simulink model "frft_qpsk_transceiver"  (R2025a)
settings: Solver=FixedStepDiscrete  StartTime=0.0  StopTime=1  RelTol=1e-3
PreLoadFcn:
  | % Add paths
  | addpath("dvb-s2/")
  | addpath("frft_filtering/")
  | addpath("gse")
  | 
  | 
  | 
  | 
  | setTxBurstLength = 10000;
  | txtmsg = ['Zynq radio HW/SW Co-design ÞÞÞÞ']; % Use only printable characters
  | 
  | %------------------------------------------------------------------------------------------------------
  | if ~isequal(size(txtmsg),[1 31])
  |     error('txtmsg must contain 31 characters');
  | end
  | 
  | [dataBits,msg] = zynqRadioHWSWQPSKgenHelloworldMsg(20); % generate 20 msgs for LUT
  | msgLUT = uint8(msg);
  | dataBitsLUT = dataBits(:);
  | Rsym                = 25e3;%1.92e6;
  | Config = zynqRadioHWSWQPSKTxRxParameters;
  | fs = Rsym*Config.SamplesPerSymbol;
  | word = [txtmsg newline];  % append a new line character to txtmsg
  | 
  | % The highest clock rate is 16 times the message character rate.
  | % As the message characters are fed at highest clock to FPGA
  | % repeat each character 16 times to maintain the message rate.
  | word = repelem(word.',16,1);
  | repeatTimes = ceil(setTxBurstLength/length(word));
  | inpData = complex(repmat(uint8(word),repeatTimes,1));
  | inUseTxBurstLength = length(inpData);
PostLoadFcn:
  | hScopeConfig = get_param([gcs '/HDL_QPSK/QPSK Tx Channel QPSK Rx/QPSK Rx/Frequency and Time Synchronizer/Symbol Synchronizer/No HDL/QPSK Receiver Eye Diagram'],'ScopeConfiguration');
  | hScopeConfig.OpenAtSimulationStart = false;
  | hScopeConfig.Visible = false;
  | clear hScopeConfig
InitFcn:
  | setTxBurstLength = 10000;
  | txtmsg = ['Zynq radio HW/SW Co-design ÞÞÞÞ']; % Use only printable characters
  | 
  | %------------------------------------------------------------------------------------------------------
  | if ~isequal(size(txtmsg),[1 31])
  |     error('txtmsg must contain 31 characters');
  | end
  | 
  | [dataBits,msg] = zynqRadioHWSWQPSKgenHelloworldMsg(20); % generate 20 msgs for LUT
  | msgLUT = uint8(msg);
  | dataBitsLUT = dataBits(:);
  | Rsym                = 25e3;%1.92e6;
  | Config = zynqRadioHWSWQPSKTxRxParameters;
  | fs = Rsym*Config.SamplesPerSymbol;
  | word = [txtmsg newline];  % append a new line character to txtmsg
  | 
  | % The highest clock rate is 16 times the message character rate.
  | % As the message characters are fed at highest clock to FPGA
  | % repeat each character 16 times to maintain the message rate.
  | word = repelem(word.',16,1);
  | repeatTimes = ceil(setTxBurstLength/length(word));
  | inpData = complex(repmat(uint8(word),repeatTimes,1));
  | inUseTxBurstLength = length(inpData);
undefined symbols (not defined in the file or in its folder): Add, dspblkCoreblockFVToolHelper, gcbh, Shift, unicode2native
libraries: hdlsllib x120, simulink x39, commseqgen3 x8, dsphdlsigops2 x4, whdledac x4, dsphdlfiltering2 x3, whdlutilities x3, dsphdlxfrm2 x2, dsphdlmathfun2 x2, commdigbbndpm3 x2, commchan3 x1, whdlmod x1
(part 2 of 5)

== system frft_qpsk_transceiver/Model Parameters/HDL_QPSK/QPSK Tx Channel QPSK Rx/QPSK Rx ==
  dataIn : Inport  OutDataTypeStr=fixdt(1,16,14)  PortDimensions=1  SampleTime=1/(Rsym*SamplesPerSymbol)
      settings: SignalType=complex
  validIn : Inport  Port=2  OutDataTypeStr=boolean  PortDimensions=1  SampleTime=1/(Rsym*SamplesPerSymbol)
  rstCS : Inport  Port=3  OutDataTypeStr=boolean  PortDimensions=1
      settings: SignalType=complex
  Automatic Gain Control : Subsystem  mask{Ref=AGCReference, LFG=AGCLoopGain}
      mask prompts: Ref "Error Detector Reference:"; LFG "Loop Filter Gain"
  Bus Creator : BusCreator  Inputs=4
  Bus Creator1 : BusCreator  Inputs=3
  Delay : Delay  DelayLength=1
  FRFT Interference Cancellation : Subsystem  Commented=on
      settings: PortSchema="{\"entries\":[{\"content\":{\"sides\":[{\"content\":{\"connectorIds\":[\"In1\",\"In2\"]},\"type\":\"ConnectorPlacement.EquallySpacedRectSide\",\"uuid\":\"50491e4b-448d-4897-93d5-82658af40e6a\"},{\"content\":{\"connectorIds\":[\"Out1\",\"Out2\"],\"side\":\"RIGHT\"},\"type\":\"ConnectorPlacement.EquallySpacedRectSide\",\"uuid\":\"92b7170a-fe32-477b-a0aa-07b62d03a88a\"},{\"content\":{\"connectorIds\":[\"In3\"],\"side\":\"TOP\"},\"type\":\"ConnectorPlacement.EquallySpacedRectSide\",\"uuid\":\"ae8eeabd-9a0c-434e-a24f-48ab553d0b87\"}]},\"type\":\"ConnectorPlacement.EquallySpacedConnector\",\"uuid\":\"9bc37ce9-ba4c-4d42-a736-75d3eb39cc46\"}],\"packageUris\":[\"http://schema.mathworks.com/mf0/Connector/R2020b\"],\"version\":\"1.0\"}"
  Frequency and Time Synchronizer : Subsystem
      settings: PortSchema="{\"entries\":[{\"content\":{\"sides\":[{\"content\":{\"connectorIds\":[\"In1\",\"In2\"]},\"type\":\"ConnectorPlacement.EquallySpacedRectSide\",\"uuid\":\"8bc6a452-5111-4806-8ca9-335cb622aea6\"},{\"content\":{\"connectorIds\":[\"Out1\",\"Out2\",\"Out3\",\"Out4\"],\"side\":\"RIGHT\"},\"type\":\"ConnectorPlacement.EquallySpacedRectSide\",\"uuid\":\"b0f43c98-f5c0-4f62-94ae-d69789942eef\"},{\"content\":{\"connectorIds\":[\"In3\",\"Out5\",\"Out6\"],\"side\":\"TOP\"},\"type\":\"ConnectorPlacement.EquallySpacedRectSide\",\"uuid\":\"427ff3b3-b896-4008-9584-d311480df763\"},{\"content\":{\"connectorIds\":[],\"side\":\"HIDDEN\"},\"type\":\"ConnectorPlacement.EquallySpacedRectSide\",\"uuid\":\"f6309498-1e43-486f-b6b5-2c6570711f8e\"}]},\"type\":\"ConnectorPlacement.EquallySpacedConnector\",\"uuid\":\"f0ce492e-c9e1-4b35-98ef-84d77b696cfe\"}],\"packageUris\":[\"http://schema.mathworks.com/mf0/Connector/R2020b\"],\"version\":\"1.0\"}"
  HDL Data Descrambler : Subsystem  Commented=on
  HDL Data Descrambler dvb : Subsystem  Commented=on
  QPSK Demodulator : Subsystem
  RRC Receive Filter : dsphdlfiltering2/Discrete FIR Filter  NumeratorSource=Property  Numerator=RRCCoef  NumeratorPrototype=[]  FilterStructure=Direct form systolic  SerializationOption=Minimum number of cycles between valid input samples  NumCycles=2  NumberOfMultipliers=2  SimulateUsing=Code generation  roundingMode=Floor  overflowMode=off  CoefficientsDataTypeStr=Inherit: Same word length as input  OutputDataTypeStr=Inherit: Same word length as input  ResetInputPort=off  HDLGlobalReset=off  CoeffMultiplier=Multiplier  UseMultForPow2Coeff=on  FrameInputSymmOptim=off
  dataOut : Outport
  ctrlOut : Outport  Port=2
  rxDiagBus : Outport  Port=3
  wires:
  Frequency and Time Synchronizer/6(normCoarseFreqEst) -> Bus Creator/2  "normCoarseFreqEst"
  QPSK Demodulator/1(dataOut) -> dataOut/1
  QPSK Demodulator/4(validOut) -> Bus Creator1/3  "validOut"
  Frequency and Time Synchronizer/1(dataOut) -> QPSK Demodulator/1(dataIn), Bus Creator/3  "QPSKConstellationPoints"
  Frequency and Time Synchronizer/4(validOut) -> QPSK Demodulator/4(validIn), Bus Creator/4  "QPSKConstellationValid"
  Frequency and Time Synchronizer/2(startOut) -> QPSK Demodulator/2(startIn)
  Frequency and Time Synchronizer/3(endOut) -> QPSK Demodulator/3(endIn)
  QPSK Demodulator/3(endOut) -> Bus Creator1/2  "endOut"
  Bus Creator1/1 -> ctrlOut/1
  RRC Receive Filter/1 -> Frequency and Time Synchronizer/1(dataIn)
  RRC Receive Filter/2 -> Frequency and Time Synchronizer/2(validIn)
  Bus Creator/1 -> Delay/1
  Frequency and Time Synchronizer/5(nSynced) -> Bus Creator/1  "nSynced"
  Automatic Gain Control/2(validOut) -> RRC Receive Filter/2
  Automatic Gain Control/1(dataOut) -> RRC Receive Filter/1
  Delay/1 -> rxDiagBus/1
  rstCS/1 -> Frequency and Time Synchronizer/3(rstCS)
  ? -> FRFT Interference Cancellation/3(rstCS)
  FRFT Interference Cancellation/1(dataOut) -> ?
  ? -> FRFT Interference Cancellation/2(validIn)
  FRFT Interference Cancellation/2(validOut) -> ?
  ? -> FRFT Interference Cancellation/1(dataIn)
  dataIn/1 -> Automatic Gain Control/1(dataIn)
  validIn/1 -> Automatic Gain Control/2(validIn)
  QPSK Demodulator/2(startOut) -> Bus Creator1/1  "startOut"

== system frft_qpsk_transceiver/Model Parameters/HDL_QPSK/QPSK Tx Channel QPSK Rx/QPSK Tx ==
  dataIn : Inport  OutDataTypeStr=boolean  PortDimensions=1
  validIn : Inport  Port=2  OutDataTypeStr=boolean  PortDimensions=1
  Bit Packetizer : Subsystem
  FEC Enabled : Constant  Value=cfg.fec_en  OutDataTypeStr=boolean
  FEC Encode : Subsystem  Commented=on
  HDL Data Scrambler_dvb : Subsystem  Commented=on
  PL Data Scrambler : Subsystem
  QPSK Modulator : Subsystem
  RRC Transmit Filter : Subsystem
  Switch{,1..3} (4 alike) : Switch  Criteria=u2 > Threshold  SaturateOnIntegerOverflow=off  InputSameDT=off
  Terminator : Terminator
  Terminator1 : Terminator
  dataOut : Outport
  validOut : Outport  Port=2
  wires:
  RRC Transmit Filter/1(dataOut) -> dataOut/1
  RRC Transmit Filter/2(validOut) -> validOut/1
  dataIn/1 -> Bit Packetizer/1(dataIn)
  validIn/1 -> Bit Packetizer/2(validIn)
  QPSK Modulator/1(dataOut) -> PL Data Scrambler/1(dataIn)  "QPSKConstellationPoints"
  QPSK Modulator/2(preambleStartOut) -> PL Data Scrambler/2(startOfPlheader)  "preambleStart"
  QPSK Modulator/3(preambleEndOut) -> PL Data Scrambler/3(endOfPlheader)  "preambleEnd"
  QPSK Modulator/4(validOut) -> PL Data Scrambler/4(validIn)  "QPSKConstellationValid"
  PL Data Scrambler/1(dataOut) -> RRC Transmit Filter/1(dataIn)  "scrambleData"
  PL Data Scrambler/2(validOut) -> RRC Transmit Filter/2(validIn)  "scrambleValid"
  Bit Packetizer/4(dataStart) -> FEC Encode/4(dataStartIn)  "FEC_DataStartIn"
  Bit Packetizer/5(dataEnd) -> FEC Encode/5(dataEndIn)  "FEC_DataEndIn"
  Bit Packetizer/1(bitsOut) -> FEC Encode/1(dataIn), Switch/3  "FEC_dataIn"
  Bit Packetizer/2(preambleStart) -> FEC Encode/2(preambleStartIn), Switch1/3  "FEC_PrStartIn"
  Bit Packetizer/3(preambleEnd) -> Switch2/3, FEC Encode/3(preambleEndIn)  "FEC_PrEndIn"
  Bit Packetizer/6(bitsValid) -> Switch3/3, FEC Encode/6(validIn)  "FEC_DataValidIn"
  FEC Encode/2(dataStartOut) -> Terminator1/1  "FEC_DataStartOut"
  FEC Encode/3(dataEndOut) -> Terminator/1  "FEC_DataEndOut"
  Switch/1 -> QPSK Modulator/1(dataIn)
  Switch1/1 -> QPSK Modulator/2(preambleStartIn)
  Switch2/1 -> QPSK Modulator/3(preambleEndIn)
  Switch3/1 -> QPSK Modulator/4(validIn)
  FEC Enabled/1 -> Switch3/2, Switch2/2, Switch1/2, Switch/2
  FEC Encode/1(dataOut) -> Switch/1  "FEC_DataOut"
  FEC Encode/4(validOut) -> Switch3/1  "FEC_DataValidOut"
  FEC Encode/6(preambleEndOut) -> Switch2/1  "FEC_PrEndOut"
  FEC Encode/5(preambleStartOut) -> Switch1/1  "FEC_PrStartOut"

== system frft_qpsk_transceiver/Model Parameters/HDL_QPSK/QPSK Tx Channel QPSK Rx/channel ==
  dataIn : Inport
  validIn : Inport  Port=2
  normalisedFreq : Inport  Port=3
  normalisedPhase : Inport  Port=4
  chirpEn : Inport  Port=5
  Add : Sum  OutDataTypeStr=Inherit: Same as first input
  Data Type Conversion : DataTypeConversion  OutDataTypeStr=fixdt(1,21,0)  ConvertRealWorld=Stored Integer (SI)  SaturateOnIntegerOverflow=off  RndMeth=Floor
  Data Type Conversion1 : DataTypeConversion  OutDataTypeStr=fixdt(1,21,0)  ConvertRealWorld=Stored Integer (SI)  SaturateOnIntegerOverflow=off  RndMeth=Floor
  Delay : Delay  DelayLength=6
  NCO HDL Optimized : dsphdlsigops2/NCO  PhaseIncrementSource=Input port  PhaseIncrement=100  PhaseOffsetSource=Input port  PhaseOffset=0  DitherSource=Property  NumDitherBits=11  SamplesPerFrame=1  LUTCompress=off  ResetAction=off  Waveform=Complex exponential  PhasePort=off  SimulateUsing=Code generation  AccumulatorWL=21  PhaseQuantization=on  NumQuantizerAccumulatorBits=14  OutputDataType=Binary point scaling  OutputWL=16  OutputFL=14
  Product : Product  OutDataTypeStr=Inherit: Same as first input
  Real-Imag to Complex : RealImagToComplex  Commented=on
  Terminator{,1..3} (4 alike) : Terminator  Commented=on
  add_chirp : MATLAB Function  Commented=on  TreatAsAtomicUnit=on  mask{fs=fs, T=16e-3, f0=0, f1=0.9*fs/2, sir=0.1}
      mask prompts: sir "SIR (Ratio)"
  dataOut : Outport
  validOut : Outport  Port=2
  wires:
  validIn/1 -> NCO HDL Optimized/3
  dataIn/1 -> Delay/1
  NCO HDL Optimized/2 -> validOut/1
  normalisedFreq/1 -> Data Type Conversion/1
  Data Type Conversion/1 -> NCO HDL Optimized/1
  NCO HDL Optimized/1 -> Product/2
  Delay/1 -> Product/1
  Data Type Conversion1/1 -> NCO HDL Optimized/2
  normalisedPhase/1 -> Data Type Conversion1/1
  chirpEn/1 -> ?
  ? -> Terminator/1  "Address_Out"
  ? -> Terminator1/1  "Address_Step_Out"
  ? -> Terminator2/1  "Address_Step_Step_Out"
  ? -> Terminator3/1  "Reset_Out"
  Product/1 -> Add/1
  Add/1 -> dataOut/1
  ? -> Real-Imag to Complex/1  "NCO_Out"
  ? -> Real-Imag to Complex/2
  Real-Imag to Complex/1 -> Add/2

== system frft_qpsk_transceiver/Model Parameters/HDL_QPSK/Subsystem/BER ==
  userBitsValid : Inport
  resetcounter : Inport  Port=2
  reset : Inport  Port=3
  userBits : Inport  Port=4
  Capture Data Bits : Subsystem
  Compare To Constant : simulink/Logic and Bit Operations/Compare To Constant  relop===  const=0  OutDataTypeStr=boolean
  Data Type Conversion1 : DataTypeConversion  OutDataTypeStr=boolean  SaturateOnIntegerOverflow=off  RndMeth=Floor
  Delay : Delay  DelayLength=1
  Delay1 : Delay  DelayLength=1
  HDL Counter : hdlsllib/Sources/HDL Counter  CountType=Free running  CountInit=0  CountStep=1  CountMax=25  CountFromType=Initial value  CountFrom=0  CountResetPort=on  CountLoadPort=off  CountEnbPort=on  CountDirPort=off  CountHitOutputPort=off  CountDataType=Unsigned  CountWordLen=32  CountFracLen=0  CountSampTime=1
  HDL Counter1 : hdlsllib/Sources/HDL Counter  CountType=Free running  CountInit=0  CountStep=1  CountMax=25  CountFromType=Initial value  CountFrom=0  CountResetPort=on  CountLoadPort=off  CountEnbPort=on  CountDirPort=off  CountHitOutputPort=off  CountDataType=Unsigned  CountWordLen=32  CountFracLen=0  CountSampTime=1
  Logical Operator : Logic  AllPortsSameDT=off  OutDataTypeStr=boolean
  Logical Operator1 : Logic  Operator=OR  AllPortsSameDT=off  OutDataTypeStr=boolean
  Relational Operator : RelationalOperator  Operator=~=  OutDataTypeStr=boolean  InputSameDT=off
  Send Payload Data : Subsystem  TreatAsAtomicUnit=on
  bitCount : Outport  VectorParamsAs1DForOutWhenUnconnected=off
  bitErrors : Outport  Port=2  VectorParamsAs1DForOutWhenUnconnected=off
  wires:
  userBits/1 -> Delay1/1
  userBitsValid/1 -> Delay/1
  resetcounter/1 -> Send Payload Data/1(rst)
  Send Payload Data/1(dataIn) -> Data Type Conversion1/1
  Data Type Conversion1/1 -> Relational Operator/2
  Relational Operator/1 -> Logical Operator/2
  Logical Operator/1 -> HDL Counter/2
  HDL Counter1/1 -> Compare To Constant/1, bitCount/1
  HDL Counter/1 -> bitErrors/1
  Compare To Constant/1 -> Logical Operator1/1
  Logical Operator1/1 -> HDL Counter/1
  Delay/1 -> Send Payload Data/2(nxtBit), Logical Operator/1, HDL Counter1/2, Capture Data Bits/Enable
  Delay1/1 -> Relational Operator/1, Capture Data Bits/1(dataOut)
  reset/1 -> HDL Counter1/1, Logical Operator1/2

== system frft_qpsk_transceiver/Model Parameters/HDL_QPSK/Subsystem/Bits to Char ==
  data : Inport
  start : Inport  Port=2
  valid : Inport  Port=3
  end : Inport  Port=4
  Add : Sum  Inputs=++|  OutDataTypeStr=uint8  AccumDataTypeStr=uint8
  Bit Shift : hdlsllib/Logic and Bit Operations/Bit Shift  mode=Shift Left Logical  N=1
  Compare To Constant : simulink/Logic and Bit Operations/Compare To Constant  relop===  const=7  OutDataTypeStr=boolean
  Data Type Conversion1 : DataTypeConversion  OutDataTypeStr=fixdt(0,1,0)  SaturateOnIntegerOverflow=off  RndMeth=Floor
  Delay{,1..4,6..7,9} (8 alike) : Delay  DelayLength=1
  Delay8 : Delay  DelayLength=13
  HDL Counter : hdlsllib/Sources/HDL Counter  CountType=Count limited  CountInit=0  CountStep=1  CountMax=7  CountFromType=Initial value  CountFrom=0  CountResetPort=on  CountLoadPort=off  CountEnbPort=on  CountDirPort=off  CountHitOutputPort=off  CountDataType=Unsigned  CountWordLen=3  CountFracLen=0  CountSampTime=1
  Logical Operator : Logic  AllPortsSameDT=off  OutDataTypeStr=boolean
  Unit Delay Enabled Resettable Synchronous : hdlsllib/Discrete/Unit Delay Enabled Resettable Synchronous  InitialCondition=0.0  SampleTime=-1
  frmStartOut : Outport
  frmEndOut : Outport  Port=2
  charOut : Outport  Port=3
  charValid : Outport  Port=4
  wires:
  data/1 -> Delay/1  "b2c_data_In"
  start/1 -> Delay7/1, HDL Counter/1  "b2c_start_In"
  Unit Delay Enabled Resettable Synchronous/1 -> Bit Shift/1
  valid/1 -> Delay1/1  "b2c_valid_In"
  Bit Shift/1 -> Add/1
  Delay/1 -> Data Type Conversion1/1
  Data Type Conversion1/1 -> Add/2
  HDL Counter/1 -> Compare To Constant/1
  Logical Operator/1 -> Unit Delay Enabled Resettable Synchronous/3, Delay2/1
  Delay1/1 -> Unit Delay Enabled Resettable Synchronous/2, Logical Operator/2, HDL Counter/2
  Compare To Constant/1 -> Logical Operator/1
  Delay2/1 -> charValid/1  "b2c_charValid_Out"
  Delay3/1 -> charOut/1  "b2c_char_Out"
  Add/1 -> Delay3/1, Unit Delay Enabled Resettable Synchronous/1
  Delay4/1 -> frmEndOut/1  "b2c_frmEnd_Out"
  end/1 -> Delay6/1
  Delay6/1 -> Delay4/1
  Delay8/1 -> Delay9/1
  Delay7/1 -> Delay8/1
  Delay9/1 -> frmStartOut/1  "b2c_frmStart_Out"

== system frft_qpsk_transceiver/Model Parameters/HDL_QPSK/QPSK Tx Channel QPSK Rx/QPSK Rx/Automatic Gain Control ==
  dataIn : Inport
  validIn : Inport  Port=2
  Data Type Duplicate : DataTypeDuplicate
  Data Type Conversion : DataTypeConversion  SaturateOnIntegerOverflow=off  RndMeth=Floor
  Delay{1..5} (5 alike) : Delay
  Error Detector : Subsystem
  Loop Filter : Subsystem
  Product : Product  OutDataTypeStr=Inherit: Same as first input
  dataOut : Outport
  validOut : Outport  Port=2
  wires:
  Data Type Conversion/1 -> Delay1/1, Data Type Duplicate/2
  Delay5/1 -> Delay3/1
  Delay3/1 -> validOut/1
  Delay4/1 -> Product/1
  Delay1/1 -> Product/2
  Loop Filter/1(gain) -> Data Type Conversion/1
  Error Detector/1(err) -> Loop Filter/1(err)
  validIn/1 -> Delay5/1
  Delay2/1 -> Error Detector/1(dataIn), dataOut/1
  dataIn/1 -> Delay4/1, Data Type Duplicate/1
  Product/1 -> Delay2/1

== system frft_qpsk_transceiver/Model Parameters/HDL_QPSK/QPSK Tx Channel QPSK Rx/QPSK Rx/FRFT Interference Cancellation ==
  dataIn : Inport
  validIn : Inport  Port=2
  rstCS : Inport  Port=3
  ChirpDDS : Subsystem
  FFT : dsphdlxfrm2/FFT  Architecture=Streaming Radix 2^2  FFTLengthSource=Property  FFTLength=1024  FFTLengthMax=1024  ComplexMultiplication=Use 4 multipliers and 2 adders  BitReversedOutput=on  BitReversedInput=off  Normalize=off  SimulateUsing=Code generation  RoundingMethod=Floor  ResetInputPort=on  StartOutputPort=on  EndOutputPort=on
  FIR FIlter : DiscreteFir  LoadFcn=dspblkCoreblockFVToolHelper(gcbh,'load');  ShowEnablePort=on
      settings: CopyFcn=dspblkCoreblockFVToolHelper(gcbh,'copy');  DeleteFcn=dspblkCoreblockFVToolHelper(gcbh,'close');  ModelCloseFcn=dspblkCoreblockFVToolHelper(gcbh,'close');  PreSaveFcn=dspblkCoreblockFVToolHelper(gcbh,'presave');  PostSaveFcn=dspblkCoreblockFVToolHelper(gcbh,'postsave');  CloseFcn=dspblkCoreblockFVToolHelper(gcbh,'close');  InputPortMap=u0,e7
  IFFT : dsphdlxfrm2/IFFT  Architecture=Streaming Radix 2^2  FFTLengthSource=Property  FFTLength=1024  FFTLengthMax=1024  ComplexMultiplication=Use 4 multipliers and 2 adders  BitReversedOutput=on  BitReversedInput=off  Normalize=on  SimulateUsing=Code generation  RoundingMethod=Floor  ResetInputPort=on  StartOutputPort=on  EndOutputPort=on
  Product : Product
  Switch : Switch  SaturateOnIntegerOverflow=off  InputSameDT=off
  dataOut : Outport
  validOut : Outport  Port=2

== system frft_qpsk_transceiver/Model Parameters/HDL_QPSK/QPSK Tx Channel QPSK Rx/QPSK Rx/Frequency and Time Synchronizer ==
  dataIn : Inport
  validIn : Inport  Port=2
  rstCS : Inport  Port=3
  Carrier Synchronizer : Subsystem
      settings: PortSchema="{\"entries\":[{\"content\":{\"sides\":[{\"content\":{\"connectorIds\":[\"In1\",\"In2\",\"In3\"]},\"type\":\"ConnectorPlacement.EquallySpacedRectSide\",\"uuid\":\"ee58e5dc-083a-48cb-b7f3-66ed8a15890f\"},{\"content\":{\"connectorIds\":[\"Out1\",\"Out2\"],\"side\":\"RIGHT\"},\"type\":\"ConnectorPlacement.EquallySpacedRectSide\",\"uuid\":\"6d121164-5065-4840-a82e-fa57a8e9650e\"},{\"content\":{\"connectorIds\":[\"In4\"],\"side\":\"TOP\"},\"type\":\"ConnectorPlacement.EquallySpacedRectSide\",\"uuid\":\"54d2b8e3-f516-4572-94a0-c914196ae8e4\"}]},\"type\":\"ConnectorPlacement.EquallySpacedConnector\",\"uuid\":\"0f2a6472-efd0-42ca-a030-ab436081b5e1\"}],\"packageUris\":[\"http://schema.mathworks.com/mf0/Connector/R2020b\"],\"version\":\"1.0\"}"
  Coarse Frequency Compensator : Subsystem
      settings: PortSchema="{\"entries\":[{\"content\":{\"sides\":[{\"content\":{\"connectorIds\":[\"In1\",\"In2\"]},\"type\":\"ConnectorPlacement.EquallySpacedRectSide\",\"uuid\":\"138aa5bd-62db-47d6-b55f-f529a6004434\"},{\"content\":{\"connectorIds\":[\"Out1\",\"Out2\",\"Out3\"],\"side\":\"RIGHT\"},\"type\":\"ConnectorPlacement.EquallySpacedRectSide\",\"uuid\":\"8e6ccec0-f736-48ab-be6d-feac886e083d\"},{\"content\":{\"connectorIds\":[\"Out4\"],\"side\":\"TOP\"},\"type\":\"ConnectorPlacement.EquallySpacedRectSide\",\"uuid\":\"d4535392-74fa-432a-a39c-b98ba26e8163\"},{\"content\":{\"side\":\"BOTTOM\"},\"type\":\"ConnectorPlacement.EquallySpacedRectSide\",\"uuid\":\"770ac6a2-7a02-4a77-858b-592982deaf6e\"}]},\"type\":\"ConnectorPlacement.EquallySpacedConnector\",\"uuid\":\"a9b944be-f88b-4ab6-a5e1-6824362eb9ca\"}],\"packageUris\":[\"http://schema.mathworks.com/mf0/Connector/R2020b\"],\"version\":\"1.0\"}"
  No HDL : Subsystem
      settings: PortSchema="{\"entries\":[{\"content\":{\"sides\":[{\"content\":{\"connectorIds\":[\"In1\",\"In2\"]},\"type\":\"ConnectorPlacement.EquallySpacedRectSide\",\"uuid\":\"df96a46d-149f-4580-adf6-e5cf26cffa9b\"},{\"content\":{\"connectorIds\":[\"In3\",\"In4\"],\"side\":\"RIGHT\"},\"type\":\"ConnectorPlacement.EquallySpacedRectSide\",\"uuid\":\"1c46d09c-cb37-4618-ac4e-e5ef50df41fb\"},{\"content\":{\"connectorIds\":[],\"side\":\"TOP\"},\"type\":\"ConnectorPlacement.EquallySpacedRectSide\",\"uuid\":\"7fe62300-46d7-4234-a31d-eecffed4f6e6\"},{\"content\":{\"connectorIds\":[],\"side\":\"BOTTOM\"},\"type\":\"ConnectorPlacement.EquallySpacedRectSide\",\"uuid\":\"05ecd563-28f5-4cfd-b718-5032a7458763\"}]},\"type\":\"ConnectorPlacement.EquallySpacedConnector\",\"uuid\":\"4b3d5859-a469-4389-9e5d-e5f07416a9a1\"}],\"packageUris\":[\"http://schema.mathworks.com/mf0/Connector/R2020b\"],\"version\":\"1.0\"}"
  PL Data Descrambler : Subsystem
  Packet Controller : Subsystem
  Phase Ambiguity Estimation and Correction : Subsystem
  Preamble Detector : Subsystem
  Symbol Synchronizer : Subsystem
  dataOut : Outport
  startOut : Outport  Port=2
  endOut : Outport  Port=3
  validOut : Outport  Port=4
  nSynced : Outport  Port=5
  normCoarseFreqEst : Outport  Port=6
  wires:
  Coarse Frequency Compensator/3(validOut) -> Carrier Synchronizer/3(validIn)
  Coarse Frequency Compensator/1(dataOut) -> Carrier Synchronizer/1(dataIn)
  Phase Ambiguity Estimation and Correction/1(dataOut) -> Packet Controller/1(dataIn)
  Phase Ambiguity Estimation and Correction/3(validOut) -> Packet Controller/3(validIn)
  Symbol Synchronizer/2(validOut) -> No HDL/2(In2), Coarse Frequency Compensator/2(validIn)
  Symbol Synchronizer/1(dataOut) -> No HDL/1(In1), Coarse Frequency Compensator/1(dataIn)
  Phase Ambiguity Estimation and Correction/2(syncPulseOut) -> Packet Controller/2(syncPulse)
  Preamble Detector/3(validOut) -> Phase Ambiguity Estimation and Correction/3(validIn)
  Preamble Detector/1(dataOut) -> Phase Ambiguity Estimation and Correction/1(dataIn)
  validIn/1 -> Symbol Synchronizer/2(validIn)
  dataIn/1 -> Symbol Synchronizer/1(dataIn)
  Coarse Frequency Compensator/2(rstCS) -> Carrier Synchronizer/2(internalRst)
  Preamble Detector/2(syncPulse) -> nSynced/1, Phase Ambiguity Estimation and Correction/2(syncPulseIn)
  Carrier Synchronizer/1(dataOut) -> No HDL/3(In3), Preamble Detector/1(dataIn)
  Carrier Synchronizer/2(validOut) -> No HDL/4(In4), Preamble Detector/2(validIn)
  Coarse Frequency Compensator/4(normalizedFreqEst) -> normCoarseFreqEst/1
  rstCS/1 -> Carrier Synchronizer/4(manualRst)
  Packet Controller/1(dataOut) -> PL Data Descrambler/1(dataIn)  "pc_dataOut"
  Packet Controller/2(startOut) -> PL Data Descrambler/2(startIn)  "pc_startOut"
  Packet Controller/3(endOut) -> PL Data Descrambler/3(endIn)  "pc_endOut"
  PL Data Descrambler/1(dataOut) -> dataOut/1  "descr_dataOut"
  PL Data Descrambler/2(startOut) -> startOut/1  "descr_startOut"
  Packet Controller/4(validOut) -> PL Data Descrambler/4(validIn)  "pc_validOut"
  PL Data Descrambler/4(validOut) -> validOut/1  "descr_validOut"
  PL Data Descrambler/3(endOut) -> endOut/1  "descr_endOut"

== system frft_qpsk_transceiver/Model Parameters/HDL_QPSK/QPSK Tx Channel QPSK Rx/QPSK Rx/HDL Data Descrambler ==
  note: HDL Data Scrambler
      | Polynomial: x^7+x^4+1
      | Initial state: [1 0 1 1 1 0 1]
  dataIn : Inport
  startIn : Inport  Port=2
  endIn : Inport  Port=3
  validIn : Inport  Port=4
  BIT_XOR : Logic  Operator=XOR  IconShape=distinctive  AllPortsSameDT=off  OutDataTypeStr=boolean
  BIT_XOR2 : Logic  Operator=XOR  IconShape=distinctive  AllPortsSameDT=off  OutDataTypeStr=boolean
  Delay{,1..7} (8 alike) : Delay  DelayLength=1
  Logical Operator : Logic  IconShape=distinctive  AllPortsSameDT=off  OutDataTypeStr=boolean
  Unit Delay Enabled Resettable Synchronous{,2..3,5,7} (5 alike) : hdlsllib/Discrete/Unit Delay Enabled Resettable Synchronous  InitialCondition=1  SampleTime=-1
  Unit Delay Enabled Resettable Synchronous1 : hdlsllib/Discrete/Unit Delay Enabled Resettable Synchronous  InitialCondition=0  SampleTime=-1
  Unit Delay Enabled Resettable Synchronous4 : hdlsllib/Discrete/Unit Delay Enabled Resettable Synchronous  InitialCondition=0  SampleTime=-1
  Unit Delay Enabled Resettable Synchronous6 : hdlsllib/Discrete/Unit Delay Enabled Resettable Synchronous  InitialCondition=0.0  SampleTime=-1
  dataOut : Outport  InitialOutput=0
  startOut : Outport  Port=2  InitialOutput=0
  endOut : Outport  Port=3  InitialOutput=0
  validOut : Outport  Port=4  InitialOutput=0
  wires:
  Delay4/1 -> validOut/1
  Delay3/1 -> dataOut/1
  endIn/1 -> Delay2/1, Unit Delay Enabled Resettable Synchronous4/3
  Logical Operator/1 -> BIT_XOR2/2
  Unit Delay Enabled Resettable Synchronous4/1 -> Logical Operator/1
  Delay1/1 -> Unit Delay Enabled Resettable Synchronous6/2, Unit Delay Enabled Resettable Synchronous2/2, Unit Delay Enabled Resettable Synchronous1/2, Unit Delay Enabled Resettable Synchronous/2, Delay4/1, Unit Delay Enabled Resettable Synchronous3/2, Unit Delay Enabled Resettable Synchronous5/2, Unit Delay Enabled Resettable Synchronous7/2
  Delay/1 -> BIT_XOR2/1
  startIn/1 -> Delay5/1, Unit Delay Enabled Resettable Synchronous4/1, Unit Delay Enabled Resettable Synchronous4/2, Unit Delay Enabled Resettable Synchronous6/3, Unit Delay Enabled Resettable Synchronous5/3, Unit Delay Enabled Resettable Synchronous1/3, Unit Delay Enabled Resettable Synchronous/3, Unit Delay Enabled Resettable Synchronous2/3, Unit Delay Enabled Resettable Synchronous3/3, Unit Delay Enabled Resettable Synchronous7/3
  dataIn/1 -> Delay/1
  validIn/1 -> Delay1/1
  BIT_XOR/1 -> Unit Delay Enabled Resettable Synchronous/1, Logical Operator/2
  Unit Delay Enabled Resettable Synchronous1/1 -> Unit Delay Enabled Resettable Synchronous2/1
  Unit Delay Enabled Resettable Synchronous2/1 -> Unit Delay Enabled Resettable Synchronous3/1
  Unit Delay Enabled Resettable Synchronous/1 -> Unit Delay Enabled Resettable Synchronous1/1
  Unit Delay Enabled Resettable Synchronous3/1 -> BIT_XOR/2, Unit Delay Enabled Resettable Synchronous5/1
  BIT_XOR2/1 -> Delay3/1
  Unit Delay Enabled Resettable Synchronous5/1 -> Unit Delay Enabled Resettable Synchronous6/1
  Unit Delay Enabled Resettable Synchronous6/1 -> Unit Delay Enabled Resettable Synchronous7/1
  Unit Delay Enabled Resettable Synchronous7/1 -> BIT_XOR/1
  Delay2/1 -> Delay6/1
  Delay5/1 -> Delay7/1
  Delay6/1 -> endOut/1
  Delay7/1 -> startOut/1

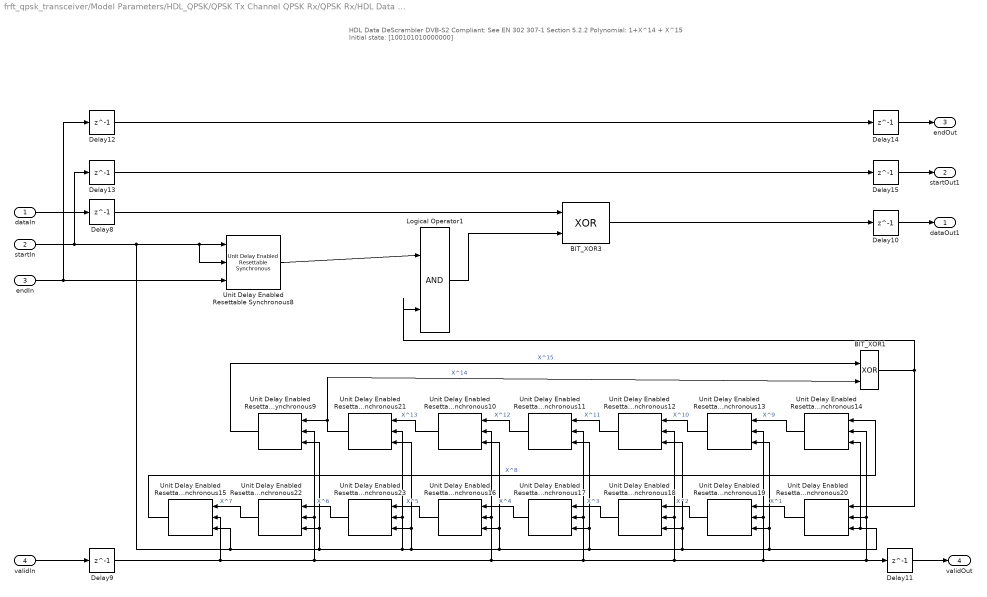
== system frft_qpsk_transceiver/Model Parameters/HDL_QPSK/QPSK Tx Channel QPSK Rx/QPSK Rx/HDL Data Descrambler dvb ==
  note: HDL Data DeScrambler
      | DVB-S2 Compliant: See EN 302 307-1 Section 5.2.2
      | Polynomial: 1+X^14 + X^15
      | Initial state: [100101010000000]
  dataIn : Inport
  startIn : Inport  Port=2
  endIn : Inport  Port=3
  validIn : Inport  Port=4
  BIT_XOR1 : Logic  Operator=XOR  IconShape=distinctive  AllPortsSameDT=off  OutDataTypeStr=boolean
  BIT_XOR3 : Logic  Operator=XOR  IconShape=distinctive  AllPortsSameDT=off  OutDataTypeStr=boolean
  Delay{8..15} (8 alike) : Delay  DelayLength=1
  Logical Operator1 : Logic  IconShape=distinctive  AllPortsSameDT=off  OutDataTypeStr=boolean
  Unit Delay Enabled Resettable Synchronous{9..14,16,18..19,21} (10 alike) : hdlsllib/Discrete/Unit Delay Enabled Resettable Synchronous  InitialCondition=0.0  SampleTime=-1
  Unit Delay Enabled Resettable Synchronous{15,17,20,23} (4 alike) : hdlsllib/Discrete/Unit Delay Enabled Resettable Synchronous  InitialCondition=1  SampleTime=-1
  Unit Delay Enabled Resettable Synchronous22 : hdlsllib/Discrete/Unit Delay Enabled Resettable Synchronous  InitialCondition=0  SampleTime=-1
  Unit Delay Enabled Resettable Synchronous8 : hdlsllib/Discrete/Unit Delay Enabled Resettable Synchronous  InitialCondition=0  SampleTime=-1
  dataOut1 : Outport  InitialOutput=0
  startOut1 : Outport  Port=2  InitialOutput=0
  endOut : Outport  Port=3  InitialOutput=0
  validOut : Outport  Port=4  InitialOutput=0
  wires:
  Delay11/1 -> validOut/1
  Unit Delay Enabled Resettable Synchronous23/1 -> Unit Delay Enabled Resettable Synchronous22/1  "X^6"
  Unit Delay Enabled Resettable Synchronous20/1 -> Unit Delay Enabled Resettable Synchronous19/1  "X^1"
  Unit Delay Enabled Resettable Synchronous21/1 -> Unit Delay Enabled Resettable Synchronous9/1, BIT_XOR1/2  "X^14"
  BIT_XOR3/1 -> Delay10/1
  Delay10/1 -> dataOut1/1
  Unit Delay Enabled Resettable Synchronous10/1 -> Unit Delay Enabled Resettable Synchronous21/1  "X^13"
  Unit Delay Enabled Resettable Synchronous22/1 -> Unit Delay Enabled Resettable Synchronous15/1  "X^7"
  Unit Delay Enabled Resettable Synchronous12/1 -> Unit Delay Enabled Resettable Synchronous11/1  "X^11"
  Unit Delay Enabled Resettable Synchronous16/1 -> Unit Delay Enabled Resettable Synchronous23/1  "X^5"
  Unit Delay Enabled Resettable Synchronous15/1 -> Unit Delay Enabled Resettable Synchronous14/1  "X^8"
  Unit Delay Enabled Resettable Synchronous17/1 -> Unit Delay Enabled Resettable Synchronous16/1  "X^4"
  Unit Delay Enabled Resettable Synchronous18/1 -> Unit Delay Enabled Resettable Synchronous17/1  "X^3"
  Unit Delay Enabled Resettable Synchronous19/1 -> Unit Delay Enabled Resettable Synchronous18/1  "X^2"
  validIn/1 -> Delay9/1
  Unit Delay Enabled Resettable Synchronous13/1 -> Unit Delay Enabled Resettable Synchronous12/1  "X^10"
  Unit Delay Enabled Resettable Synchronous9/1 -> BIT_XOR1/1  "X^15"
  Unit Delay Enabled Resettable Synchronous14/1 -> Unit Delay Enabled Resettable Synchronous13/1  "X^9"
  Unit Delay Enabled Resettable Synchronous11/1 -> Unit Delay Enabled Resettable Synchronous10/1  "X^12"
  dataIn/1 -> Delay8/1
  Delay8/1 -> BIT_XOR3/1
  BIT_XOR1/1 -> Unit Delay Enabled Resettable Synchronous20/1, Logical Operator1/2
  Delay9/1 -> Unit Delay Enabled Resettable Synchronous15/2, Unit Delay Enabled Resettable Synchronous22/2, Unit Delay Enabled Resettable Synchronous9/2, Unit Delay Enabled Resettable Synchronous10/2, Unit Delay Enabled Resettable Synchronous16/2, Unit Delay Enabled Resettable Synchronous12/2, Unit Delay Enabled Resettable Synchronous18/2, Unit Delay Enabled Resettable Synchronous13/2, Unit Delay Enabled Resettable Synchronous19/2, Unit Delay Enabled Resettable Synchronous14/2, Unit Delay Enabled Resettable Synchronous20/2, Delay11/1, Unit Delay Enabled Resettable Synchronous11/2, Unit Delay Enabled Resettable Synchronous17/2
  Unit Delay Enabled Resettable Synchronous8/1 -> Logical Operator1/1
  Logical Operator1/1 -> BIT_XOR3/2
  endIn/1 -> Delay12/1, Unit Delay Enabled Resettable Synchronous8/3
  Delay12/1 -> Delay14/1
  Delay13/1 -> Delay15/1
  startIn/1 -> Delay13/1, Unit Delay Enabled Resettable Synchronous15/3, Unit Delay Enabled Resettable Synchronous9/3, Unit Delay Enabled Resettable Synchronous22/3, Unit Delay Enabled Resettable Synchronous21/2, Unit Delay Enabled Resettable Synchronous23/2, Unit Delay Enabled Resettable Synchronous21/3, Unit Delay Enabled Resettable Synchronous23/3, Unit Delay Enabled Resettable Synchronous10/3, Unit Delay Enabled Resettable Synchronous16/3, Unit Delay Enabled Resettable Synchronous18/3, Unit Delay Enabled Resettable Synchronous12/3, Unit Delay Enabled Resettable Synchronous19/3, Unit Delay Enabled Resettable Synchronous13/3, Unit Delay Enabled Resettable Synchronous14/3, Unit Delay Enabled Resettable Synchronous20/3, Unit Delay Enabled Resettable Synchronous17/3, Unit Delay Enabled Resettable Synchronous11/3, Unit Delay Enabled Resettable Synchronous8/2, Unit Delay Enabled Resettable Synchronous8/1
  Delay14/1 -> endOut/1
  Delay15/1 -> startOut1/1

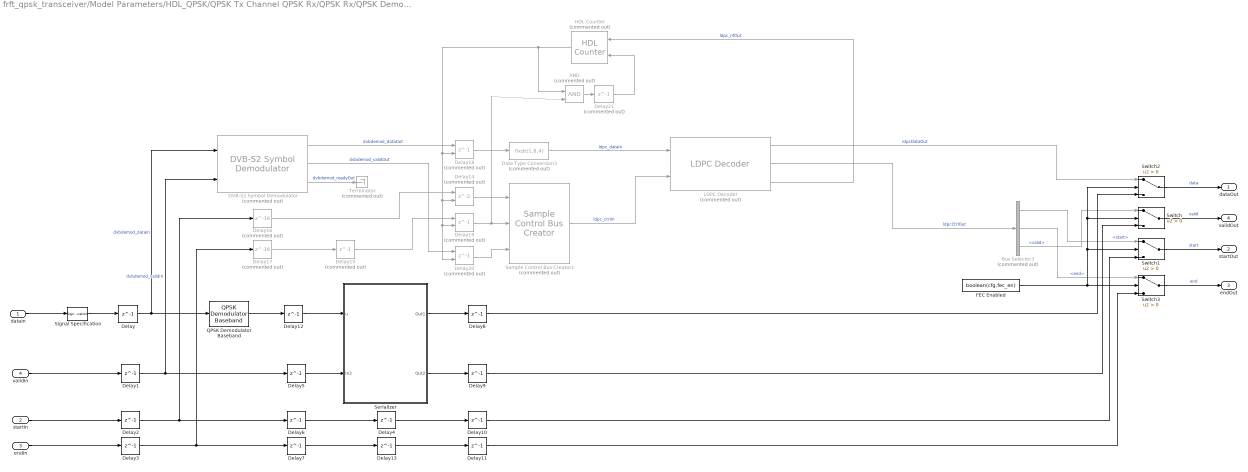
== system frft_qpsk_transceiver/Model Parameters/HDL_QPSK/QPSK Tx Channel QPSK Rx/QPSK Rx/QPSK Demodulator ==
  dataIn : Inport
  startIn : Inport  Port=2
  endIn : Inport  Port=3
  validIn : Inport  Port=4
  AND : Logic  Commented=on  IconShape=distinctive  AllPortsSameDT=off  OutDataTypeStr=boolean
  Bus Selector3 : BusSelector  Commented=on  OutputSignals=start,end,valid
  DVB-S2 Symbol Demodulator : whdlmod/DVB-S2 Symbol Demodulator  Commented=on  ModulationSourceParams=Property  ModulationScheme=QPSK  CodeRateAPSK=3/4  DecisionType=Approximate log-likelihood ratio  OutputType=Scalar  UnitAveragePower=off  EnbNoiseVar=off  SimulateUsing=Code generation
  Data Type Conversion3 : DataTypeConversion  Commented=on  OutDataTypeStr=fixdt(1,8,4)  RndMeth=Floor
  Delay{,1..13} (14 alike) : Delay  DelayLength=1
  Delay14 : Delay  Commented=on  ShowEnablePort=on
      settings: InputPortMap=u0,e6
  Delay15 : Delay  Commented=on  DelayLength=1
  Delay16 : Delay  Commented=on  DelayLength=16
  Delay17 : Delay  Commented=on  DelayLength=16
  Delay18 : Delay  Commented=on  DelayLength=1  ShowEnablePort=on
      settings: InputPortMap=u0,e6
  Delay19 : Delay  Commented=on  DelayLength=1  ShowEnablePort=on
      settings: InputPortMap=u0,e6
  Delay20 : Delay  Commented=on  DelayLength=1  ShowEnablePort=on
      settings: InputPortMap=u0,e6
  Delay21 : Delay  Commented=on  DelayLength=1
  FEC Enabled : Constant  Value=boolean(cfg.fec_en)
  HDL Counter : hdlsllib/Sources/HDL Counter  Commented=on  CountType=Count limited  CountInit=1  CountStep=-1  CountMax=0  CountFromType=Initial value  CountFrom=1  CountResetPort=on  CountLoadPort=off  CountEnbPort=on  CountDirPort=off  CountHitOutputPort=off  CountDataType=Unsigned  CountWordLen=1  CountFracLen=0  CountSampTime=1
  LDPC Decoder : whdledac/LDPC Decoder  Commented=on  ParityCheckMatrix=cfg.parityCheckMatrix  BlockSize=cfg.blockSize  Algorithm=Min-sum  ScalingFactor=alpha  Termination=Max  SpecifyInputs=Property  NumIterations=8  MaxNumIterations=8  ParityCheckStatus=off  SimulateUsing=Code generation
  QPSK Demodulator Baseband : commdigbbndpm3/QPSK Demodulator Baseband  OutType=Bit  DecType=Hard decision  VarSource=Dialog  Variance=1  Dec=Gray  Ph=pi/4  outDtype1=boolean  outDtype2=Inherit via internal rule  derotateFactorWordLen=16  derotateFactorDataTypeStr=Inherit: Same word length as input  derotateFactorLastDataTypeStr=Inherit: Same word length as input
  Sample Control Bus Creator1 : whdlutilities/Sample Control Bus Creator  Commented=on
  Serializer : Subsystem
  Signal Specification : SignalSpecification  Dimensions=1
  Switch{,1..3} (4 alike) : Switch  Criteria=u2 > Threshold  SaturateOnIntegerOverflow=off  InputSameDT=off
  Terminator : Terminator  Commented=on
  dataOut : Outport
  startOut : Outport  Port=2
  endOut : Outport  Port=3
  validOut : Outport  Port=4
  wires:
  Delay/1 -> DVB-S2 Symbol Demodulator/1, QPSK Demodulator Baseband/1  "dvbdemod_dataIn"
  Delay1/1 -> Delay5/1, DVB-S2 Symbol Demodulator/2  "dvbdemod_validIn"
  Delay6/1 -> Delay4/1
  Delay7/1 -> Delay13/1
  Delay2/1 -> Delay6/1, Delay16/1
  Signal Specification/1 -> Delay/1
  QPSK Demodulator Baseband/1 -> Delay12/1
  Delay5/1 -> Serializer/2(In2)
  Delay12/1 -> Serializer/1(u)
  Delay4/1 -> Delay10/1
  Delay13/1 -> Delay11/1
  Serializer/1(Out1) -> Delay8/1
  Serializer/2(Out2) -> Delay9/1
  dataIn/1 -> Signal Specification/1
  validIn/1 -> Delay1/1
  startIn/1 -> Delay2/1
  endIn/1 -> Delay3/1
  DVB-S2 Symbol Demodulator/1 -> Delay18/1  "dvbdemod_dataOut"
  LDPC Decoder/1 -> Switch2/1  "ldpcDataOut"
  LDPC Decoder/3 -> HDL Counter/1  "ldpc_nfOut"
  Data Type Conversion3/1 -> LDPC Decoder/1  "ldpc_dataIn"
  Sample Control Bus Creator1/1 -> LDPC Decoder/2  "ldpc_ctrlIn"
  DVB-S2 Symbol Demodulator/3 -> Terminator/1  "dvbdemod_readyOut"
  Delay3/1 -> Delay17/1, Delay7/1
  Delay14/1 -> Sample Control Bus Creator1/1
  Delay15/1 -> Delay19/1
  Delay16/1 -> Delay14/1
  Delay17/1 -> Delay15/1
  Delay18/1 -> Data Type Conversion3/1
  Delay19/1 -> AND/2, Sample Control Bus Creator1/2
  DVB-S2 Symbol Demodulator/2 -> Delay20/1  "dvbdemod_validOut"
  Delay20/1 -> Sample Control Bus Creator1/3
  HDL Counter/1 -> AND/1, Delay20/2, Delay19/2, Delay14/2, Delay18/2
  AND/1 -> Delay21/1
  Delay21/1 -> HDL Counter/2
  LDPC Decoder/2 -> Bus Selector3/1  "ldpcCtrlOut"
  Switch2/1 -> dataOut/1  "data"
  Switch/1 -> validOut/1  "valid"
  Switch1/1 -> startOut/1  "start"
  Switch3/1 -> endOut/1  "end"
  Bus Selector3/1 -> Switch1/1  "<start>"
  Bus Selector3/2 -> Switch3/1  "<end>"
  Bus Selector3/3 -> Switch/1  "<valid>"
  FEC Enabled/1 -> Switch3/2, Switch1/2, Switch/2, Switch2/2
  Delay8/1 -> Switch2/3
  Delay9/1 -> Switch/3
  Delay10/1 -> Switch1/3
  Delay11/1 -> Switch3/3

== system frft_qpsk_transceiver/Model Parameters/HDL_QPSK/QPSK Tx Channel QPSK Rx/QPSK Tx/Bit Packetizer ==
  dataIn : Inport
  validIn : Inport  Port=2
  Compare To Constant : hdlsllib/Logic and Bit Operations/Compare To Constant  relop===  const=length(Preamble)  OutDataTypeStr=boolean
  Compare To Constant1 : hdlsllib/Logic and Bit Operations/Compare To Constant  relop===  const=bitsPerPacket - 1  OutDataTypeStr=boolean
  Compare To Constant2 : hdlsllib/Logic and Bit Operations/Compare To Constant  relop=>=  const=length(Preamble)  OutDataTypeStr=boolean
  Compare To Constant3 : hdlsllib/Logic and Bit Operations/Compare To Constant  relop===  const=0  OutDataTypeStr=boolean
  Compare To Constant4 : hdlsllib/Logic and Bit Operations/Compare To Constant  relop===  const=length(Preamble)-1  OutDataTypeStr=boolean
  Data Bits FIFO : Subsystem
  Data Type Conversion : DataTypeConversion  OutDataTypeStr=boolean  SaturateOnIntegerOverflow=off  RndMeth=Floor
  HDL Counter : hdlsllib/Sources/HDL Counter  CountType=Count limited  CountInit=0  CountStep=1  CountMax=1  CountFromType=Initial value  CountFrom=0  CountResetPort=off  CountLoadPort=off  CountEnbPort=on  CountDirPort=off  CountHitOutputPort=off  CountDataType=Unsigned  CountWordLen=1  CountFracLen=0  CountSampTime=1
  Logical Operator{,1,3..4} (4 alike) : Logic  AllPortsSameDT=off  OutDataTypeStr=boolean
  Logical Operator2 : Logic  Operator=NOT  AllPortsSameDT=off  OutDataTypeStr=boolean
  Preamble Bits Generator : Subsystem
  Switch : Switch  Criteria=u2 ~= 0  SaturateOnIntegerOverflow=off  InputSameDT=off
  Terminator : Terminator
  bitsOut : Outport
  preambleStart : Outport  Port=2
  preambleEnd : Outport  Port=3
  dataStart : Outport  Port=4
  dataEnd : Outport  Port=5
  bitsValid : Outport  Port=6
  wires:
  dataIn/1 -> Data Bits FIFO/1(data)
  validIn/1 -> Data Bits FIFO/2(push)
  Compare To Constant/1 -> Logical Operator/1
  Compare To Constant1/1 -> Logical Operator1/2
  Logical Operator/1 -> dataStart/1
  Logical Operator1/1 -> dataEnd/1
  Data Bits FIFO/5(fullRAM) -> Logical Operator2/1
  Logical Operator2/1 -> HDL Counter/1
  Data Bits FIFO/1(dataOut) -> Switch/1
  Data Bits FIFO/3(sampleCount) -> Compare To Constant/1, Compare To Constant4/1, Compare To Constant3/1, Compare To Constant1/1, Compare To Constant2/1, Preamble Bits Generator/2(sampleCount)
  Data Bits FIFO/4(sampleCountValid) -> bitsValid/1, Logical Operator/2, Logical Operator4/1, Logical Operator3/1, Logical Operator1/1, Preamble Bits Generator/3(sampleCountValid)
  Data Bits FIFO/2(activeFrame) -> Preamble Bits Generator/1(activeFrame)
  Preamble Bits Generator/1(preambleBits) -> Switch/3
  Compare To Constant2/1 -> Switch/2
  Switch/1 -> bitsOut/1
  HDL Counter/1 -> Data Type Conversion/1
  Data Type Conversion/1 -> Terminator/1
  Compare To Constant3/1 -> Logical Operator3/2
  Compare To Constant4/1 -> Logical Operator4/2
  Logical Operator3/1 -> preambleStart/1
  Logical Operator4/1 -> preambleEnd/1

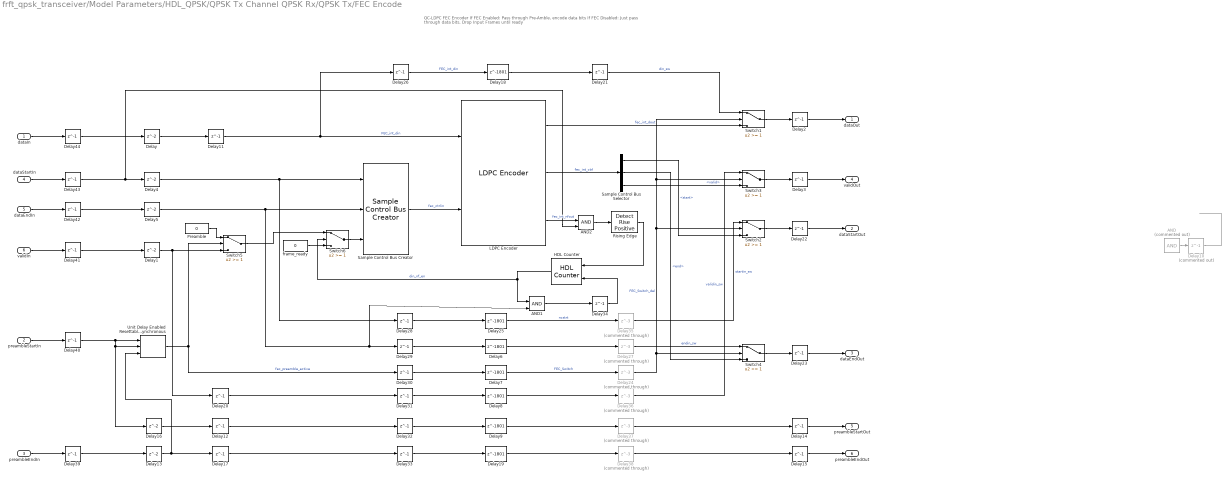
== system frft_qpsk_transceiver/Model Parameters/HDL_QPSK/QPSK Tx Channel QPSK Rx/QPSK Tx/FEC Encode ==
  note: QC-LDPC FEC Encoder
      |
      | If FEC Enabled: Pass through Pre-Amble, encode data bits
      | If FEC Disabled: Just pass through data bits.
      | Drop Input Frames until ready
  dataIn : Inport
  preambleStartIn : Inport  Port=2
  preambleEndIn : Inport  Port=3
  dataStartIn : Inport  Port=4
  dataEndIn : Inport  Port=5
  validIn : Inport  Port=6
  AND : Logic  Commented=on  IconShape=distinctive  AllPortsSameDT=off  OutDataTypeStr=boolean
  AND1 : Logic  IconShape=distinctive  AllPortsSameDT=off  OutDataTypeStr=boolean
  AND2 : Logic  IconShape=distinctive  AllPortsSameDT=off  OutDataTypeStr=boolean
  Delay{,1,4..5,13,16} (6 alike) : Delay
  Delay10 : Delay  Commented=on  DelayLength=1
  Delay{2..3,11..12,14..15,17,20..23,26,28..34,39..44} (25 alike) : Delay  DelayLength=1
  Delay{6..9,18..19,25} (7 alike) : Delay  DelayLength=1801
  Delay{24,27,35..38} (6 alike) : Delay  Commented=through  DelayLength=3
  HDL Counter : hdlsllib/Sources/HDL Counter  CountType=Count limited  CountInit=1  CountStep=-1  CountMax=0  CountFromType=Initial value  CountFrom=1  CountResetPort=on  CountLoadPort=off  CountEnbPort=on  CountDirPort=off  CountHitOutputPort=off  CountDataType=Unsigned  CountWordLen=1  CountFracLen=0  CountSampTime=1
  LDPC Encoder : whdledac/LDPC Encoder  ParityCheckMatrix=cfg.parityCheckMatrix  BlockSize=cfg.blockSize  SimulateUsing=Code generation
  Preamble : Constant  Value=0  OutDataTypeStr=boolean
  Rising Edge : hdlsllib/Logic and Bit Operations/Detect Rise Positive  vinit=0  OutDataTypeStr=boolean
  Sample Control Bus Creator : whdlutilities/Sample Control Bus Creator
  Sample Control Bus Selector : BusSelector  OutputSignals=start,end,valid
  Switch{1..6} (6 alike) : Switch  Threshold=1  SaturateOnIntegerOverflow=off  InputSameDT=off
  Unit Delay Enabled Resettable Synchronous : hdlsllib/Discrete/Unit Delay Enabled Resettable Synchronous  InitialCondition=0.0  SampleTime=-1
  frame_ready : Constant  Value=0  OutDataTypeStr=boolean
  dataOut : Outport
  dataStartOut : Outport  Port=2
  dataEndOut : Outport  Port=3
  validOut : Outport  Port=4
  preambleStartOut : Outport  Port=5
  preambleEndOut : Outport  Port=6
  wires:
  dataIn/1 -> Delay44/1
  validIn/1 -> Delay41/1
  Delay2/1 -> dataOut/1
  Delay3/1 -> validOut/1
  Delay14/1 -> preambleStartOut/1
  Delay15/1 -> preambleEndOut/1
  dataStartIn/1 -> Delay43/1
  dataEndIn/1 -> Delay42/1
  preambleStartIn/1 -> Delay40/1
  Unit Delay Enabled Resettable Synchronous/1 -> Delay30/1, Switch5/2  "fec_preamble_active"
  Delay1/1 -> Delay20/1, Switch5/3
  Delay5/1 -> AND1/2, Delay29/1, Sample Control Bus Creator/2
  Delay/1 -> Delay11/1
  Delay11/1 -> Delay26/1, LDPC Encoder/1  "FEC_int_din"
  preambleEndIn/1 -> Delay39/1
  Delay13/1 -> Delay17/1, Unit Delay Enabled Resettable Synchronous/3
  Delay16/1 -> Delay12/1
  Delay12/1 -> Delay32/1
  Delay17/1 -> Delay33/1
  Delay9/1 -> Delay37/1
  Delay19/1 -> Delay38/1
  Delay20/1 -> Delay31/1
  LDPC Encoder/2 -> Sample Control Bus Selector/1  "fec_int_ctrl"
  Sample Control Bus Selector/2 -> Switch4/3  "<end>"
  Sample Control Bus Selector/1 -> Switch2/3  "<start>"
  Switch3/1 -> Delay3/1
  Switch1/1 -> Delay2/1
  Delay18/1 -> Delay21/1
  LDPC Encoder/1 -> Switch1/3  "fec_int_dout"
  Sample Control Bus Selector/3 -> Switch3/3  "<valid>"
  Delay8/1 -> Delay36/1
  Delay7/1 -> Delay24/1  "FEC_Switch"
  Switch4/1 -> Delay23/1
  Delay23/1 -> dataEndOut/1
  Delay22/1 -> dataStartOut/1
  Switch2/1 -> Delay22/1
  Delay25/1 -> Delay35/1  "ncstrt"
  Delay6/1 -> Delay27/1
  Preamble/1 -> Switch5/1
  Sample Control Bus Creator/1 -> LDPC Encoder/2  "fec_ctrlin"
  ? -> AND/1
  Delay10/1 -> ?
  ? -> AND/2
  AND/1 -> Delay10/1
  Delay26/1 -> Delay18/1  "FEC_int_din"
  Delay28/1 -> Delay25/1
  Delay30/1 -> Delay7/1
  Delay31/1 -> Delay8/1
  Delay32/1 -> Delay9/1
  Delay33/1 -> Delay19/1
  HDL Counter/1 -> AND1/1, Switch6/2  "din_nf_en"
  Delay34/1 -> HDL Counter/2
  AND1/1 -> Delay34/1
  Delay29/1 -> Delay6/1
  Rising Edge/1 -> HDL Counter/1
  Switch6/1 -> Sample Control Bus Creator/3
  frame_ready/1 -> Switch6/3
  Switch5/1 -> Switch6/1
  LDPC Encoder/3 -> AND2/1  "fec_int_nfout"
  AND2/1 -> Rising Edge/1
  Delay4/1 -> Delay28/1, Sample Control Bus Creator/1
  Delay21/1 -> Switch1/1  "din_sw"
  Delay24/1 -> Switch2/2, Switch3/2, Switch1/2, Switch4/2  "FEC_Switch_del"
  Delay27/1 -> Switch4/1  "endin_sw"
  Delay35/1 -> Switch2/1  "startin_sw"
  Delay36/1 -> Switch3/1  "validin_sw"
  Delay37/1 -> Delay14/1
  Delay38/1 -> Delay15/1
  Delay39/1 -> Delay13/1
  Delay40/1 -> Unit Delay Enabled Resettable Synchronous/1, Unit Delay Enabled Resettable Synchronous/2, Delay16/1
  Delay41/1 -> Delay1/1
  Delay42/1 -> Delay5/1
  Delay43/1 -> AND2/2, Delay4/1
  Delay44/1 -> Delay/1
